simulink model "All_Four_wheel_PID23"  (R2026a)
settings: Solver=ode4  FixedStep=0.001
libraries: simulink x1
settings Model: Creator=dell

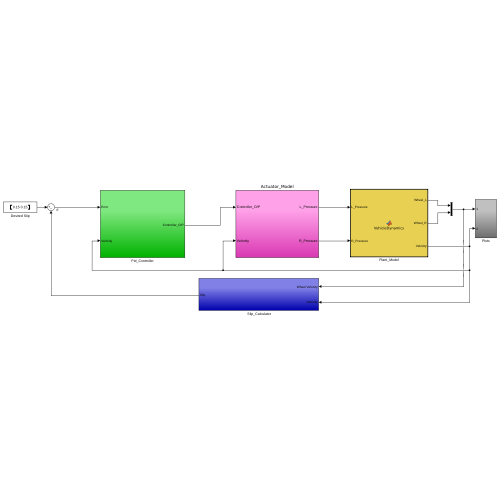
[thumbnail: Simulink's stored preview of the top-level diagram]
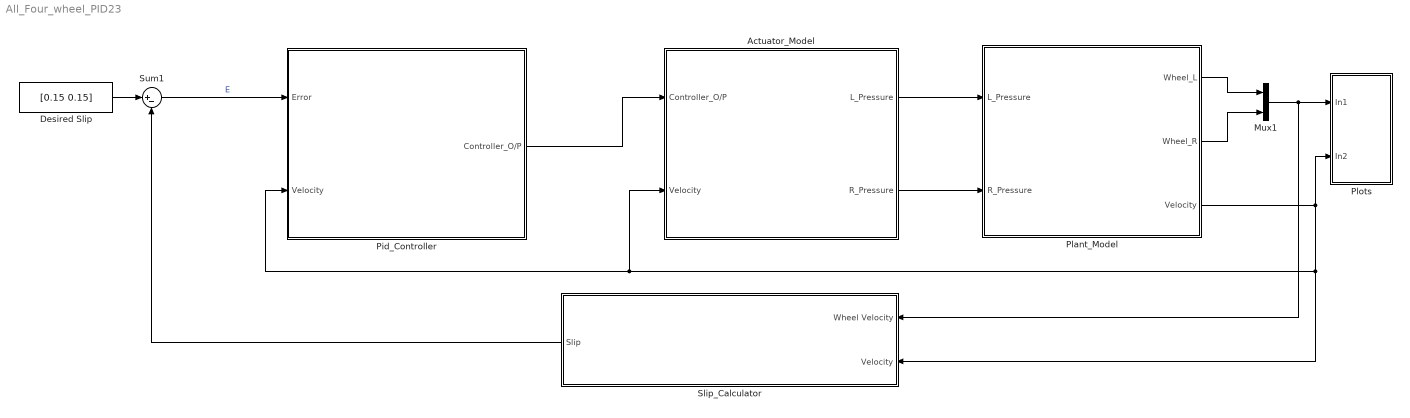
== system All_Four_wheel_PID23 ==
  " Slip_Calculator" : Subsystem
  Actuator_Model : Subsystem
  "Desired Slip " : Constant  Value=[0.15 0.15]
  Mux1 : Mux  Inputs=2
  Pid_Controller : Subsystem
  Plant_Model : MATLAB Function  TreatAsAtomicUnit=on
  Plots : Subsystem
  Sum1 : Sum  Inputs=|+-
  wires:
  "Desired Slip "/1 -> Sum1/1
  Mux1/1 -> " Slip_Calculator"/1(Wheel Velocity), Plots/1(In1)
  " Slip_Calculator"/1(Slip) -> Sum1/2
  Plant_Model/1(Wheel_L) -> Mux1/1
  Plant_Model/2(Wheel_R) -> Mux1/2
  Plant_Model/3(Velocity) -> " Slip_Calculator"/2(Velocity), Pid_Controller/2(Velocity), Actuator_Model/2(Velocity), Plots/2(In2)
  Actuator_Model/1(L_Pressure) -> Plant_Model/1(L_Pressure)
  Actuator_Model/2(R_Pressure) -> Plant_Model/2(R_Pressure)
  Pid_Controller/1(Controller_O/P) -> Actuator_Model/1(Controller_O/P)
  Sum1/1 -> Pid_Controller/1(Error)  "E"

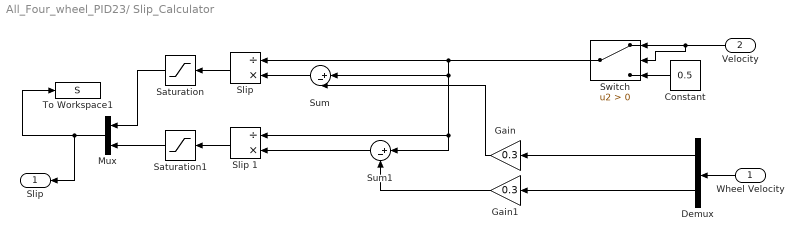
== system All_Four_wheel_PID23/ Slip_Calculator ==
  Wheel Velocity : Inport
  Velocity : Inport  Port=2
  Constant : Constant  Value=0.5
  Demux : Demux  Outputs=2
  Gain : Gain  Gain=0.3
  Gain1 : Gain  Gain=0.3
  Mux : Mux  Inputs=2
  Saturation : Saturate  UpperLimit=1  LowerLimit=0
  Saturation1 : Saturate  UpperLimit=1  LowerLimit=0
  "Slip " : Product  Inputs=/*  InputSameDT=on  SaturateOnIntegerOverflow=on  OutDataTypeStr=Inherit: Same as first input
  Slip 1 : Product  Inputs=/*  InputSameDT=on  SaturateOnIntegerOverflow=on  OutDataTypeStr=Inherit: Same as first input
  Sum : Sum  Inputs=|+-
  Sum1 : Sum  Inputs=|+-
  Switch : Switch  Criteria=u2 > Threshold  SaturateOnIntegerOverflow=off  InputSameDT=off
  To Workspace1 : ToWorkspace  VariableName=S  SaveFormat=Structure With Time  SampleTime=0.002
  Slip : Outport
  wires:
  Sum/1 -> "Slip "/2
  "Slip "/1 -> Saturation/1
  Slip 1/1 -> Saturation1/1
  Saturation1/1 -> Mux/2
  Sum1/1 -> Slip 1/2
  Wheel Velocity/1 -> Demux/1
  Saturation/1 -> Mux/1
  Mux/1 -> To Workspace1/1, Slip/1
  Demux/1 -> Gain/1
  Gain/1 -> Sum/2
  Demux/2 -> Gain1/1
  Gain1/1 -> Sum1/2
  Switch/1 -> Sum1/1, Slip 1/1, Sum/1, "Slip "/1
  Velocity/1 -> Switch/2, Switch/1
  Constant/1 -> Switch/3

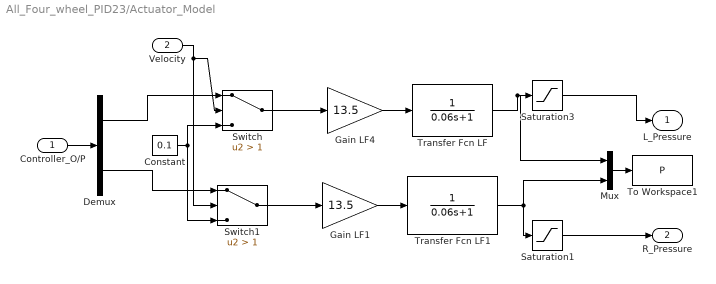
== system All_Four_wheel_PID23/Actuator_Model ==
  Controller_O/P : Inport
  Velocity : Inport  Port=2
  Constant : Constant  Value=0.1
  Demux : Demux  Outputs=2
  Gain LF1 : Gain  Gain=13.5  SaturateOnIntegerOverflow=on  OutDataTypeStr=Inherit: Same as input  ParamDataTypeStr=Inherit: Same as input
  Gain LF4 : Gain  Gain=13.5  SaturateOnIntegerOverflow=on  OutDataTypeStr=Inherit: Same as input  ParamDataTypeStr=Inherit: Same as input
  Mux : Mux  Inputs=2
  Saturation1 : Saturate  UpperLimit=1  LowerLimit=0
  Saturation3 : Saturate  UpperLimit=1  LowerLimit=0
  Switch : Switch  Criteria=u2 > Threshold  Threshold=1  SaturateOnIntegerOverflow=off  InputSameDT=off
  Switch1 : Switch  Criteria=u2 > Threshold  Threshold=1  SaturateOnIntegerOverflow=off  InputSameDT=off
  To Workspace1 : ToWorkspace  VariableName=P  SaveFormat=Structure With Time  SampleTime=0.002
  Transfer Fcn LF : TransferFcn  Denominator=[0.06 1]
  Transfer Fcn LF1 : TransferFcn  Denominator=[0.06 1]
  L_Pressure : Outport  InitialOutput=0
  R_Pressure : Outport  Port=2
  wires:
  Transfer Fcn LF/1 -> Saturation3/1, Mux/1
  Transfer Fcn LF1/1 -> Mux/2, Saturation1/1
  Mux/1 -> To Workspace1/1
  Gain LF4/1 -> Transfer Fcn LF/1
  Gain LF1/1 -> Transfer Fcn LF1/1
  Controller_O/P/1 -> Demux/1
  Velocity/1 -> Switch1/2, Switch/2
  Constant/1 -> Switch1/3, Switch/3
  Demux/1 -> Switch/1
  Switch/1 -> Gain LF4/1
  Demux/2 -> Switch1/1
  Switch1/1 -> Gain LF1/1
  Saturation3/1 -> L_Pressure/1
  Saturation1/1 -> R_Pressure/1

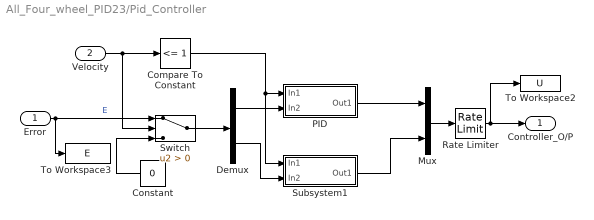
== system All_Four_wheel_PID23/Pid_Controller ==
  Error : Inport
  Velocity : Inport  Port=2
  Compare To Constant : simulink/Logic and Bit Operations/Compare To Constant  relop=<=  const=1  OutDataTypeStr=boolean
  Constant : Constant  Value=0
  Demux : Demux  Outputs=2
  Mux : Mux  Inputs=2
  PID : Subsystem
  Rate Limiter : RateLimiter  RisingSlewLimit=16.67  FallingSlewLimit=-16.67  SampleTimeMode=inherited
  Subsystem1 : Subsystem
  Switch : Switch  Criteria=u2 > Threshold  SaturateOnIntegerOverflow=off  InputSameDT=off
  To Workspace2 : ToWorkspace  VariableName=U  SaveFormat=Structure With Time  SampleTime=0.002
  To Workspace3 : ToWorkspace  VariableName=E  SaveFormat=Structure With Time  SampleTime=0.002
  Controller_O/P : Outport
  wires:
  Velocity/1 -> Compare To Constant/1, Switch/2
  Compare To Constant/1 -> Subsystem1/1(In1), PID/1(In1)
  Demux/1 -> PID/2(In2)
  PID/1(Out1) -> Mux/1
  Subsystem1/1(Out1) -> Mux/2
  Demux/2 -> Subsystem1/2(In2)
  Mux/1 -> Rate Limiter/1
  Rate Limiter/1 -> Controller_O/P/1, To Workspace2/1
  Switch/1 -> Demux/1
  Constant/1 -> Switch/3
  Error/1 -> Switch/1, To Workspace3/1  "E"

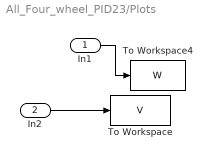
== system All_Four_wheel_PID23/Plots ==
  In1 : Inport
  In2 : Inport  Port=2
  To Workspace : ToWorkspace  VariableName=V  SaveFormat=Structure With Time  SampleTime=0.002
  To Workspace4 : ToWorkspace  VariableName=W  SaveFormat=Structure With Time  SampleTime=0.002
  wires:
  In1/1 -> To Workspace4/1
  In2/1 -> To Workspace/1

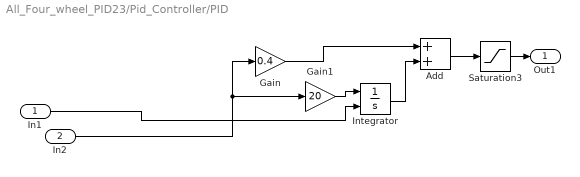
== system All_Four_wheel_PID23/Pid_Controller/PID ==
  In1 : Inport
  In2 : Inport  Port=2
  Add : Sum
  Gain : Gain  Gain=0.4
  Gain1 : Gain  Gain=20
  Integrator : Integrator  ExternalReset=level
  Saturation3 : Saturate  UpperLimit=1  LowerLimit=0
  Out1 : Outport
  wires:
  Saturation3/1 -> Out1/1
  Gain1/1 -> Integrator/1
  In2/1 -> Gain/1, Gain1/1
  Add/1 -> Saturation3/1
  Gain/1 -> Add/1
  Integrator/1 -> Add/2
  In1/1 -> Integrator/2

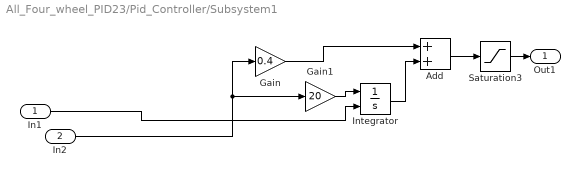
== system All_Four_wheel_PID23/Pid_Controller/Subsystem1 ==
  In1 : Inport
  In2 : Inport  Port=2
  Add : Sum
  Gain : Gain  Gain=0.4
  Gain1 : Gain  Gain=20
  Integrator : Integrator  ExternalReset=level
  Saturation3 : Saturate  UpperLimit=1  LowerLimit=0
  Out1 : Outport
  wires:
  In1/1 -> Integrator/2
  Integrator/1 -> Add/2
  Gain/1 -> Add/1
  Add/1 -> Saturation3/1
  In2/1 -> Gain1/1, Gain/1
  Gain1/1 -> Integrator/1
  Saturation3/1 -> Out1/1

== matlab function All_Four_wheel_PID23/Plant_Model ==
  settings: updateMethod=DISCRETE
  data: L_Pressure input; R_Pressure input; Wheel_L output; Wheel_R output; Velocity output
function [Wheel_L, Wheel_R, Velocity] = VehicleDynamics(L_Pressure, R_Pressure)

% Vehicle parameters
r   = 0.30;     % wheel radius (m)
m   = 1500;     % UAV mass (kg)
I   = 2.0;      % wheel inertia (kg.m^2)
Kb  = 75;       % brake gain
b_w = 1.0;      % wheel damping
dt  = 0.001;    % simulation time step (s)
g   = 9.81;     % gravity (m/s^2)

Wheel_max = 100;
Wheel_min = 0;
Vel_max   = 30;
Vel_min   = 0;

% Initialization
persistent Wheel_L_prev Wheel_R_prev Velocity_prev
if isempty(Wheel_L_prev)

    
    Velocity_prev = 20;    %m/s
    Wheel_L_prev = Velocity_prev / r;   % rad/s
    Wheel_R_prev = Velocity_prev / r;   % rad/s

end

% Brake torques 
Tbr = [Kb*L_Pressure, Kb*R_Pressure];

% Wheel rotational dynamics
Wheel_prev = [Wheel_L_prev, Wheel_R_prev];
Wheel = Wheel_prev + ((-Tbr - b_w*Wheel_prev)/I)*dt;
Wheel = min(max(Wheel, Wheel_min), Wheel_max);

Wheel_L = Wheel(1);
Wheel_R = Wheel(2);

% Wheel slip calculation
slip_vec = max((Velocity_prev - Wheel*r) / max(Velocity_prev, 0.1), 0);
slip_vec = min(slip_vec, 1);

% Tyre friction coefficient
mu_vec = 1.0 - 0.25 * slip_vec;
mu_vec = max(mu_vec, 0);
mu_vec = min(mu_vec, 1);

% Longitudinal braking forces
NormalLoad = 0.8 * m * g / 2;       
Fxf_vec = mu_vec .* NormalLoad;

% Vehicle longitudinal dynamics
Fbr_total = sum(Fxf_vec);      
a = -Fbr_total / m;            

Velocity = Velocity_prev + a * dt;
Velocity = max(min(Velocity, Vel_max), Vel_min);

% Updated states
Wheel_L_prev = Wheel_L;
Wheel_R_prev = Wheel_R;
Velocity_prev = Velocity;

end
